simulink model "tank_based_bi_teleop_pf"  (R2020b)
settings: Solver=VariableStepAuto  StartTime=0.0  StopTime=4.0  RelTol=1e-3
values from neighbouring files (symbols this model uses):
  A = 1    [four_channel_bilateral_teleoperation_kalman_params.m]    (also in four_channel_bilateral_teleoperation_params.m; kalman_test.m = [1 Ts Ts^2/2; 0 1 Ts; 0 0 1]; recursive_estimation.m = [1 Ts Ts^2/2; 0 1 Ts; 0 0 1]; scattering_based_bi_teleop_pf_kalman_params.m)
  Be = 100    [four_channel_bilateral_teleoperation_architecture_params.m]    (also in four_channel_bilateral_teleoperation_kalman_params.m = 0; four_channel_bilateral_teleoperation_params.m = 0; scattering_based_bi_teleop_pf_kalman_params.m = 10; scattering_based_bi_teleop_pf_params.m = 10)
  Bh = 70    [four_channel_bilateral_teleoperation_architecture_params.m]    (also in four_channel_bilateral_teleoperation_kalman_params.m; four_channel_bilateral_teleoperation_params.m; scattering_based_bi_teleop_pf_kalman_params.m = 1.5; scattering_based_bi_teleop_pf_params.m = 1.5)
  Bm = 1    [four_channel_bilateral_teleoperation_architecture_params.m]    (also in four_channel_bilateral_teleoperation_kalman_params.m = 0.8; four_channel_bilateral_teleoperation_params.m = 0.8; scattering_based_bi_teleop_pf_kalman_params.m = 0; scattering_based_bi_teleop_pp_kalman_params.m = 15)
  Bs = 1    [four_channel_bilateral_teleoperation_architecture_params.m]    (also in four_channel_bilateral_teleoperation_kalman_params.m = 3.2; four_channel_bilateral_teleoperation_params.m = 3.2; scattering_based_bi_teleop_pf_kalman_params.m = 40; scattering_based_bi_teleop_pf_params.m = 3)
  Dh = 500    [four_channel_bilateral_teleoperation_kalman_params.m]    (also in four_channel_bilateral_teleoperation_params.m = 100; scattering_based_bi_teleop_pf_kalman_params.m = 0; scattering_based_bi_teleop_pf_params.m = 17; scattering_based_bi_teleop_pp_kalman_params.m = 0)
  Dm = 5    [four_channel_bilateral_teleoperation_architecture_params.m]    (also in four_channel_bilateral_teleoperation_kalman_params.m = 0; four_channel_bilateral_teleoperation_params.m = 0; scattering_based_bi_teleop_pf_kalman_params.m = 0; scattering_based_bi_teleop_pf_params.m = 0)
  Ds = 10    [four_channel_bilateral_teleoperation_architecture_params.m]    (also in four_channel_bilateral_teleoperation_kalman_params.m = 0; four_channel_bilateral_teleoperation_params.m = 0; scattering_based_bi_teleop_pf_kalman_params.m = 0; scattering_based_bi_teleop_pf_params.m = 0)
  Fc = 1    [four_channel_bilateral_teleoperation_kalman_params.m]    (also in four_channel_bilateral_teleoperation_params.m; kalman_test.m = 10; scattering_based_bi_teleop_pf_kalman_params.m = 0.1; scattering_based_bi_teleop_pf_params.m)
  Fip = 1    [four_channel_bilateral_teleoperation_kalman_params.m]    (also in four_channel_bilateral_teleoperation_params.m; scattering_based_bi_teleop_pf_kalman_params.m = 5; scattering_based_bi_teleop_pf_params.m; scattering_based_bi_teleop_pp_kalman_params.m = 5)
  Je = 0    [four_channel_bilateral_teleoperation_architecture_params.m]    (also in four_channel_bilateral_teleoperation_kalman_params.m; four_channel_bilateral_teleoperation_params.m; scattering_based_bi_teleop_pf_kalman_params.m; scattering_based_bi_teleop_pf_params.m)
  Jh = 0.5    [four_channel_bilateral_teleoperation_architecture_params.m]    (also in four_channel_bilateral_teleoperation_kalman_params.m; four_channel_bilateral_teleoperation_params.m; scattering_based_bi_teleop_pf_kalman_params.m = 0; scattering_based_bi_teleop_pf_params.m = 0.05)
  Ke = 200    [four_channel_bilateral_teleoperation_architecture_params.m]    (also in four_channel_bilateral_teleoperation_kalman_params.m = 50; four_channel_bilateral_teleoperation_params.m = 50; scattering_based_bi_teleop_pf_kalman_params.m; scattering_based_bi_teleop_pf_params.m)
  Kh = 2000    [four_channel_bilateral_teleoperation_architecture_params.m]    (also in four_channel_bilateral_teleoperation_kalman_params.m; four_channel_bilateral_teleoperation_params.m; scattering_based_bi_teleop_pf_kalman_params.m = 1; scattering_based_bi_teleop_pf_params.m = 0)
  Km = 1    [four_channel_bilateral_teleoperation_architecture_params.m]    (also in four_channel_bilateral_teleoperation_kalman_params.m; four_channel_bilateral_teleoperation_params.m; scattering_based_bi_teleop_pf_kalman_params.m = 0; scattering_based_bi_teleop_pp_kalman_params.m = 10)
  Ks = 1    [four_channel_bilateral_teleoperation_architecture_params.m]    (also in four_channel_bilateral_teleoperation_kalman_params.m = 4; four_channel_bilateral_teleoperation_params.m = 4; scattering_based_bi_teleop_pf_kalman_params.m = 50; scattering_based_bi_teleop_pf_params.m = 110)
  Mm = 0.5    [four_channel_bilateral_teleoperation_architecture_params.m]    (also in four_channel_bilateral_teleoperation_kalman_params.m; four_channel_bilateral_teleoperation_params.m; scattering_based_bi_teleop_pf_kalman_params.m; scattering_based_bi_teleop_pf_params.m)
  Ms = 2    [four_channel_bilateral_teleoperation_architecture_params.m]    (also in four_channel_bilateral_teleoperation_kalman_params.m; four_channel_bilateral_teleoperation_params.m; scattering_based_bi_teleop_pf_kalman_params.m; scattering_based_bi_teleop_pf_params.m)
  Ph = 2000    [four_channel_bilateral_teleoperation_kalman_params.m]    (also in four_channel_bilateral_teleoperation_params.m = 20100; scattering_based_bi_teleop_pf_kalman_params.m = 5; scattering_based_bi_teleop_pf_params.m = 23; scattering_based_bi_teleop_pp_kalman_params.m = 6)
  Ts = 0.001    [four_channel_bilateral_teleoperation_kalman_params.m]    (also in four_channel_bilateral_teleoperation_params.m; kalman_test.m; recursive_estimation.m; scattering_based_bi_teleop_pf_kalman_params.m)
undefined symbols (not defined in the file or in its folder): tau
libraries: simulink x2
settings Model: Creator=anuj  LastModifiedBy=filippo

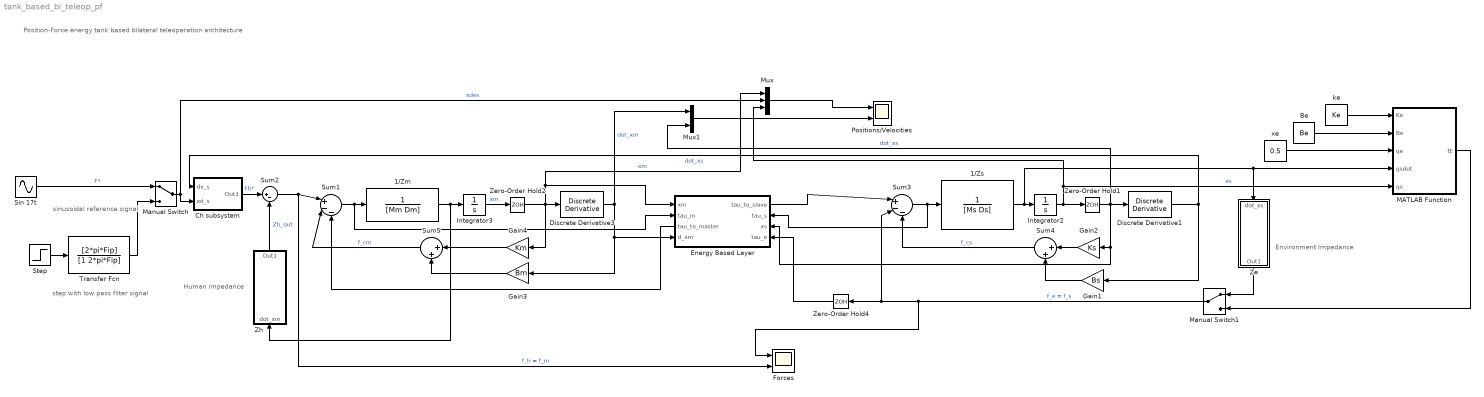
== system tank_based_bi_teleop_pf ==
  note: Position-Force energy tank based bilateral teleoperation architecture
  note: Environment Impedance
  note: Human impedance
  note: sinusoidal reference signal
  note: step with low pass filter signal
  1/Zm : TransferFcn  Denominator=[Mm Dm]
  1/Zs : TransferFcn  Denominator=[Ms Ds]
  Be : Constant  Value=Be
  Ch subsystem : Subsystem
  Discrete Derivative1 : simulink/Discrete/Discrete Derivative  gainval=1.0  ICPrevScaledInput=0.0  OutMin=[]  OutMax=[]  OutDataType=fixdt(1, 16)  OutScaling=2^-10  DoSatur=off
  Discrete Derivative3 : simulink/Discrete/Discrete Derivative  gainval=1.0  ICPrevScaledInput=0.0  OutMin=[]  OutMax=[]  OutDataType=fixdt(1, 16)  OutScaling=2^-10  DoSatur=off
  Energy Based Layer : Subsystem
      settings: PortSchema="{\"entries\":[{\"content\":{\"sides\":[{\"content\":{\"connectorIds\":[\"In1\",\"In2\",\"Out2\",\"In3\"]},\"type\":\"ConnectorPlacement.EquallySpacedRectSide\",\"uuid\":\"721fd75b-d64f-459b-a3fd-bbe3848745a1\"},{\"content\":{\"connectorIds\":[\"Out1\",\"In4\",\"In5\",\"In6\"],\"side\":\"RIGHT\"},\"type\":\"ConnectorPlacement.EquallySpacedRectSide\",\"uuid\":\"fbbe53d8-b5f9-4b89-bc3e-da0a725f4cb9\"},{\"content\":{\"connectorIds\":[],\"side\":\"TOP\"},\"type\":\"ConnectorPlacement.EquallySpacedRectSide\",\"uuid\":\"8cd4d438-c323-4c6b-8da9-ae64782b16ea\"},{\"content\":{\"connectorIds\":[],\"side\":\"HIDDEN\"},\"type\":\"ConnectorPlacement.EquallySpacedRectSide\",\"uuid\":\"3c4adbce-c957-4479-b649-6006afc34fa2\"}]},\"type\":\"ConnectorPlacement.EquallySpacedConnector\",\"uuid\":\"ae1c0201-3e75-47b3-8045-db2a4ffaac12\"}],\"packageUris\":[\"http://schema.mathworks.com/mf0/Connector/R2020b\"],\"version\":\"1.0\"}"
  Forces : Scope  NumInputPorts=2
  Gain1 : Gain  Gain=Bs
  Gain2 : Gain  Gain=Ks
  Gain3 : Gain  Gain=Bm
  Gain4 : Gain  Gain=Km
  Integrator2 : Integrator
  Integrator3 : Integrator
  MATLAB Function : MATLAB Function  TreatAsAtomicUnit=on
  Manual Switch : ManualSwitch
  Manual Switch1 : ManualSwitch
  Mux : Mux  Inputs=3
  Mux1 : Mux  Inputs=2
  Positions/Velocities : Scope  NumInputPorts=2
  Sin 17t : Sin  Amplitude=A  Frequency=2*pi*Fc  SampleTime=0
  Step : Step  After=A  SampleTime=0
  Sum1 : Sum  Inputs=|+--
  Sum2 : Sum  Inputs=|+-
  Sum3 : Sum  Inputs=|+--
  Sum4 : Sum  Inputs=|++
  Sum5 : Sum  Inputs=|++
  Transfer Fcn : TransferFcn  Numerator=[2*pi*Fip]  Denominator=[1 2*pi*Fip]
  Ze : Subsystem
  Zero-Order Hold1 : ZeroOrderHold  SampleTime=Ts
  Zero-Order Hold2 : ZeroOrderHold  SampleTime=Ts
  Zero-Order Hold4 : ZeroOrderHold  SampleTime=Ts
  Zh : Subsystem
  ke : Constant  Value=Ke
  xe : Constant  Value=0.5
  wires:
  Sum2/1 -> Forces/2, Sum1/1  "f_h = f_m"
  1/Zm/1 -> Integrator3/1, Zh/1(dot_xm)
  Sum1/1 -> Energy Based Layer/2(tau_m), 1/Zm/1
  Energy Based Layer/2(tau_to_master) -> Sum1/3
  Sum3/1 -> Energy Based Layer/4(tau_s), 1/Zs/1
  Manual Switch1/1 -> Forces/1, Sum3/2, Zero-Order Hold4/1  "f_e = f_s"
  Be/1 -> MATLAB Function/2(Be)
  xe/1 -> MATLAB Function/3(qe)
  ke/1 -> MATLAB Function/1(Ke)
  Transfer Fcn/1 -> Manual Switch/2
  Step/1 -> Transfer Fcn/1
  Sin 17t/1 -> Manual Switch/1  "F*"
  Energy Based Layer/1(tau_to_slave) -> Sum3/1
  Zh/1(Out1) -> Sum2/2  "Zh_out"
  Sum5/1 -> Sum1/2  "f_cm"
  Sum4/1 -> Sum3/3  "f_cs"
  Discrete Derivative1/1 -> Gain1/1, Ch subsystem/1(dx_s)  "dot_xs"
  1/Zs/1 -> Integrator2/1, Ze/1(dot_xs), MATLAB Function/4(qsdot)
  Integrator2/1 -> Zero-Order Hold1/1, Mux/3, MATLAB Function/5(qs)  "xs"
  Gain2/1 -> Sum4/1
  Gain1/1 -> Sum4/2
  Zero-Order Hold1/1 -> Mux1/2, Gain2/1, Energy Based Layer/5(xs), Discrete Derivative1/1  "dot_xs"
  Integrator3/1 -> Zero-Order Hold2/1  "xm"
  Gain4/1 -> Sum5/1
  Gain3/1 -> Sum5/2
  Discrete Derivative3/1 -> Energy Based Layer/3(d_xm), Gain3/1, Mux1/1  "dot_xm"
  Zero-Order Hold2/1 -> Energy Based Layer/1(xm), Mux/1, Gain4/1, Discrete Derivative3/1  "xm"
  Zero-Order Hold4/1 -> Energy Based Layer/6(tau_e)
  Ze/1(Out1) -> Manual Switch1/1
  MATLAB Function/1(fE) -> Manual Switch1/2
  Mux1/1 -> Positions/Velocities/2
  Mux/1 -> Positions/Velocities/1
  Manual Switch/1 -> Mux/2, Ch subsystem/2(xd_s)  "xdes"
  Ch subsystem/1(Out1) -> Sum2/1  "Fh*"

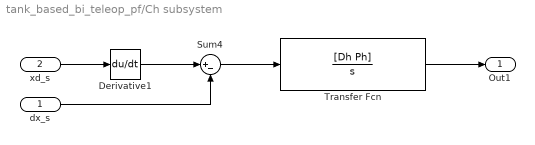
== system tank_based_bi_teleop_pf/Ch subsystem ==
  dx_s : Inport
  xd_s : Inport  Port=2
  Derivative1 : Derivative
  Sum4 : Sum  Inputs=|+-
  Transfer Fcn : TransferFcn  Numerator=[Dh Ph]  Denominator=[1 0]
  Out1 : Outport
  wires:
  dx_s/1 -> Sum4/2
  Derivative1/1 -> Sum4/1
  xd_s/1 -> Derivative1/1
  Sum4/1 -> Transfer Fcn/1
  Transfer Fcn/1 -> Out1/1

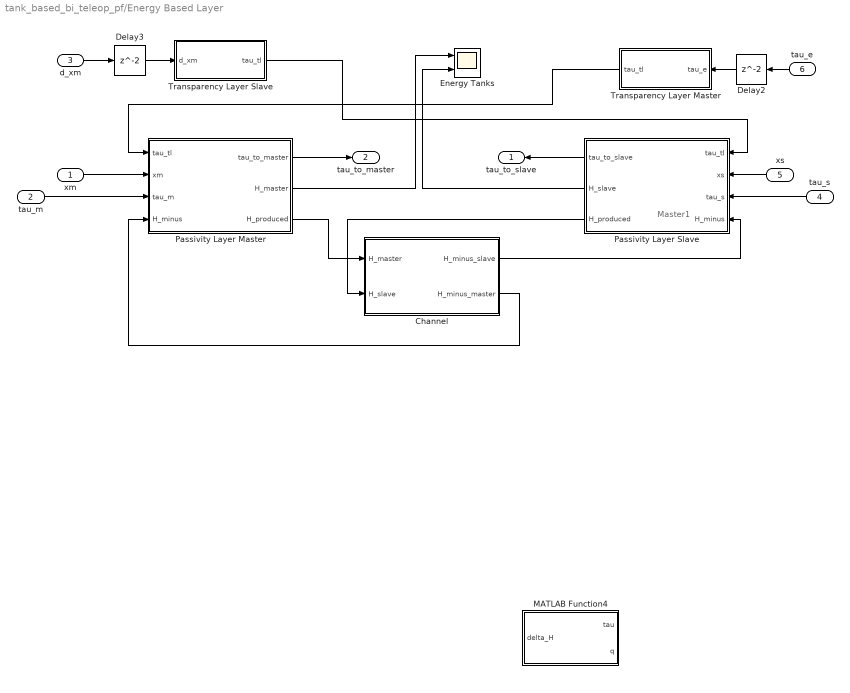
== system tank_based_bi_teleop_pf/Energy Based Layer ==
  note: Master1
  xm : Inport
  tau_m : Inport  Port=2
  d_xm : Inport  Port=3
  tau_s : Inport  Port=4
  xs : Inport  Port=5
  tau_e : Inport  Port=6
  Channel : Subsystem
  Delay2 : Delay
  Delay3 : Delay
  Energy Tanks : Scope  NumInputPorts=2
  MATLAB Function4 : MATLAB Function  TreatAsAtomicUnit=on
  Passivity Layer Master : Subsystem
  "Passivity Layer Slave " : Subsystem
  Transparency Layer Master : Subsystem
  Transparency Layer Slave : Subsystem
  tau_to_slave : Outport
  tau_to_master : Outport  Port=2
  wires:
  tau_e/1 -> Delay2/1
  Delay2/1 -> Transparency Layer Master/1(tau_e)
  d_xm/1 -> Delay3/1
  Delay3/1 -> Transparency Layer Slave/1(d_xm)
  tau_m/1 -> Passivity Layer Master/3(tau_m)
  xm/1 -> Passivity Layer Master/2(xm)
  tau_s/1 -> "Passivity Layer Slave "/3(tau_s)
  xs/1 -> "Passivity Layer Slave "/2(xs)
  "Passivity Layer Slave "/1(tau_to_slave) -> tau_to_slave/1
  Passivity Layer Master/1(tau_to_master) -> tau_to_master/1
  Passivity Layer Master/2(H_master) -> Energy Tanks/1
  "Passivity Layer Slave "/2(H_slave) -> Energy Tanks/2
  Passivity Layer Master/3(H_produced) -> Channel/1(H_master)
  "Passivity Layer Slave "/3(H_produced) -> Channel/2(H_slave)
  Channel/1(H_minus_slave) -> "Passivity Layer Slave "/4(H_minus)
  Channel/2(H_minus_master) -> Passivity Layer Master/4(H_minus)
  Transparency Layer Slave/1(tau_tl) -> "Passivity Layer Slave "/1(tau_tl)
  Transparency Layer Master/1(tau_tl) -> Passivity Layer Master/1(tau_tl)

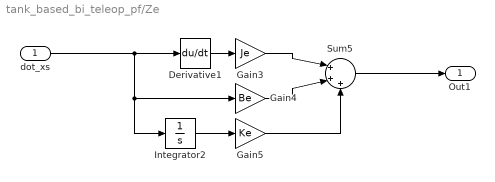
== system tank_based_bi_teleop_pf/Ze ==
  dot_xs : Inport
  Derivative1 : Derivative
  Gain3 : Gain  Gain=Je
  Gain4 : Gain  Gain=Be
  Gain5 : Gain  Gain=Ke
  Integrator2 : Integrator
  Sum5 : Sum  Inputs=|+++
  Out1 : Outport
  wires:
  Gain4/1 -> Sum5/2
  Gain3/1 -> Sum5/1
  Gain5/1 -> Sum5/3
  Sum5/1 -> Out1/1
  Integrator2/1 -> Gain5/1
  dot_xs/1 -> Integrator2/1, Gain4/1, Derivative1/1
  Derivative1/1 -> Gain3/1

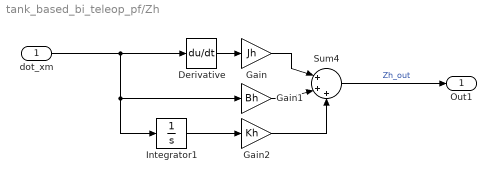
== system tank_based_bi_teleop_pf/Zh ==
  dot_xm : Inport
  Derivative : Derivative
  Gain : Gain  Gain=Jh
  Gain1 : Gain  Gain=Bh
  Gain2 : Gain  Gain=Kh
  Integrator1 : Integrator
  Sum4 : Sum  Inputs=|+++
  Out1 : Outport
  wires:
  Derivative/1 -> Gain/1
  Integrator1/1 -> Gain2/1
  Gain2/1 -> Sum4/3
  Gain1/1 -> Sum4/2
  Gain/1 -> Sum4/1
  Sum4/1 -> Out1/1  "Zh_out"
  dot_xm/1 -> Gain1/1, Integrator1/1, Derivative/1

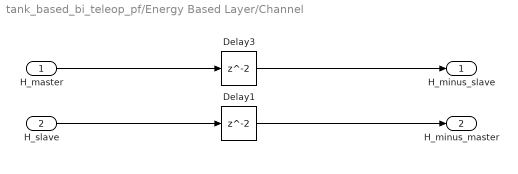
== system tank_based_bi_teleop_pf/Energy Based Layer/Channel ==
  H_master : Inport
  H_slave : Inport  Port=2
  Delay1 : Delay
  Delay3 : Delay
  H_minus_slave : Outport
  H_minus_master : Outport  Port=2
  wires:
  H_master/1 -> Delay3/1
  H_slave/1 -> Delay1/1
  Delay3/1 -> H_minus_slave/1
  Delay1/1 -> H_minus_master/1

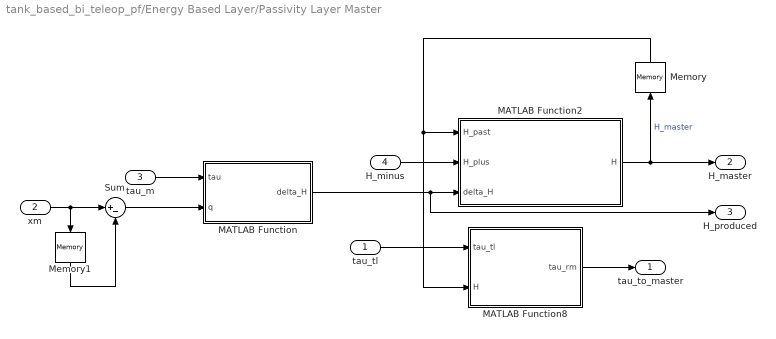
== system tank_based_bi_teleop_pf/Energy Based Layer/Passivity Layer Master ==
  tau_tl : Inport
  xm : Inport  Port=2
  tau_m : Inport  Port=3
  H_minus : Inport  Port=4
  MATLAB Function : MATLAB Function  TreatAsAtomicUnit=on
  MATLAB Function2 : MATLAB Function  TreatAsAtomicUnit=on
  MATLAB Function8 : MATLAB Function  TreatAsAtomicUnit=on
  Memory : Memory
  Memory1 : Memory
  Sum : Sum  Inputs=|+-
  tau_to_master : Outport
  H_master : Outport  Port=2
  H_produced : Outport  Port=3
  wires:
  MATLAB Function2/1(H) -> H_master/1, Memory/1  "H_master"
  tau_m/1 -> MATLAB Function/1(tau)
  Memory/1 -> MATLAB Function8/2(H), MATLAB Function2/1(H_past)
  MATLAB Function/1(delta_H) -> H_produced/1, MATLAB Function2/3(delta_H)
  xm/1 -> Sum/1, Memory1/1
  tau_tl/1 -> MATLAB Function8/1(tau_tl)
  H_minus/1 -> MATLAB Function2/2(H_plus)
  Memory1/1 -> Sum/2
  Sum/1 -> MATLAB Function/2(q)
  MATLAB Function8/1(tau_rm) -> tau_to_master/1

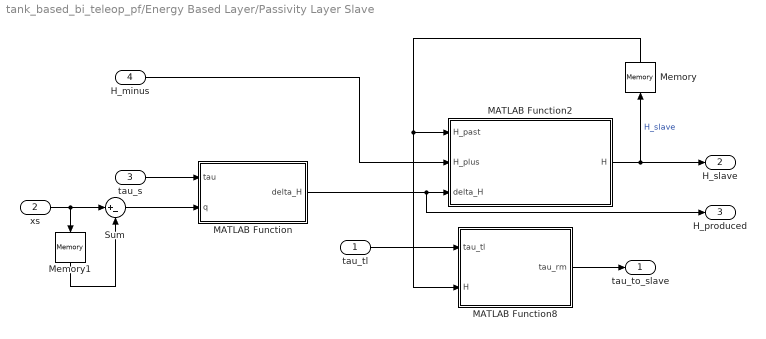
== system tank_based_bi_teleop_pf/Energy Based Layer/Passivity Layer Slave  ==
  tau_tl : Inport
  xs : Inport  Port=2
  tau_s : Inport  Port=3
  H_minus : Inport  Port=4
  MATLAB Function : MATLAB Function  TreatAsAtomicUnit=on
  MATLAB Function2 : MATLAB Function  TreatAsAtomicUnit=on
  MATLAB Function8 : MATLAB Function  TreatAsAtomicUnit=on
  Memory : Memory
  Memory1 : Memory
  Sum : Sum  Inputs=|+-
  tau_to_slave : Outport
  H_slave : Outport  Port=2
  H_produced : Outport  Port=3
  wires:
  MATLAB Function2/1(H) -> H_slave/1, Memory/1  "H_slave"
  tau_s/1 -> MATLAB Function/1(tau)
  Memory/1 -> MATLAB Function8/2(H), MATLAB Function2/1(H_past)
  MATLAB Function/1(delta_H) -> H_produced/1, MATLAB Function2/3(delta_H)
  MATLAB Function8/1(tau_rm) -> tau_to_slave/1
  tau_tl/1 -> MATLAB Function8/1(tau_tl)
  H_minus/1 -> MATLAB Function2/2(H_plus)
  Sum/1 -> MATLAB Function/2(q)
  xs/1 -> Sum/1, Memory1/1
  Memory1/1 -> Sum/2

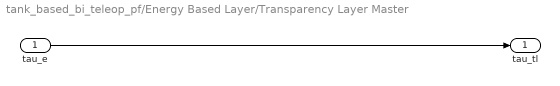
== system tank_based_bi_teleop_pf/Energy Based Layer/Transparency Layer Master ==
  tau_e : Inport
  tau_tl : Outport
  wires:
  tau_e/1 -> tau_tl/1

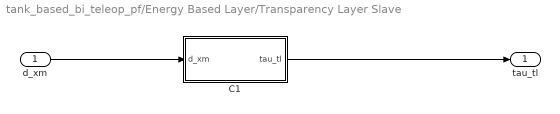
== system tank_based_bi_teleop_pf/Energy Based Layer/Transparency Layer Slave ==
  d_xm : Inport
  C1 : Subsystem
  tau_tl : Outport
  wires:
  d_xm/1 -> C1/1(d_xm)
  C1/1(tau_tl) -> tau_tl/1

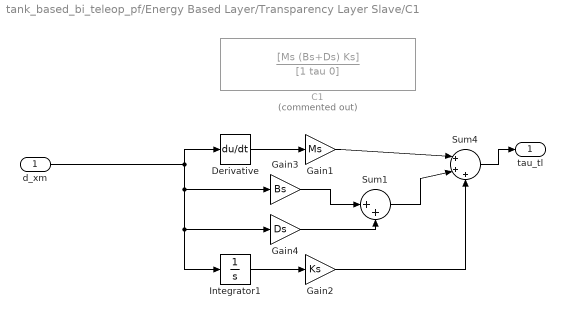
== system tank_based_bi_teleop_pf/Energy Based Layer/Transparency Layer Slave/C1 ==
  d_xm : Inport
  C1 : TransferFcn  Commented=on  Numerator=[Ms (Bs+Ds) Ks]  Denominator=[1 tau 0]
  Derivative : Derivative
  Gain1 : Gain  Gain=Ms
  Gain2 : Gain  Gain=Ks
  Gain3 : Gain  Gain=Bs
  Gain4 : Gain  Gain=Ds
  Integrator1 : Integrator
  Sum1 : Sum  Inputs=|++
  Sum4 : Sum  Inputs=|+++
  tau_tl : Outport
  wires:
  Sum4/1 -> tau_tl/1
  Gain1/1 -> Sum4/1
  Integrator1/1 -> Gain2/1
  d_xm/1 -> Derivative/1, Gain3/1, Integrator1/1, Gain4/1
  Gain2/1 -> Sum4/3
  Sum1/1 -> Sum4/2
  Gain4/1 -> Sum1/2
  Gain3/1 -> Sum1/1
  Derivative/1 -> Gain1/1

== matlab function tank_based_bi_teleop_pf/Energy Based Layer/Passivity Layer Slave /MATLAB Function ==
  data: tau input; delta_H output; q input
function delta_H = delta_H(tau, q)
    delta_H = tau*q;
end

== matlab function tank_based_bi_teleop_pf/MATLAB Function ==
  data: Ke input; fE output; Be input; qe input; qsdot input; qs input
function fE = environment(Ke, Be, qe, qsdot, qs)
    if qs > qe
        fE = Ke * (qs - qe) + Be * qsdot; % Plot both contributions Ke and Be
    else
        fE = 0;
    end
end

== matlab function tank_based_bi_teleop_pf/Energy Based Layer/Passivity Layer Slave /MATLAB Function2 ==
  data: H output; H_past input; H_plus input; delta_H input
function H = EnergyTank(H_past, H_plus, delta_H)
    H = H_past + H_plus - delta_H;
end

== matlab function tank_based_bi_teleop_pf/Energy Based Layer/Passivity Layer Slave /MATLAB Function8 ==
  data: tau_tl input; tau_rm output; H input
function tau_rm = tau_saturation(tau_tl, H)
    tau_max1 = tau_tl;
    if H <= 0 
       tau_max1 = 0;
    end
    
    tau_rm = sign(tau_tl)*min(abs(tau_tl), tau_max1);
end

== matlab function tank_based_bi_teleop_pf/Energy Based Layer/MATLAB Function4 ==
  data: tau input; delta_H output; q input
function delta_H = delta_H(tau, q)
    delta_H = tau*q;
end

== matlab function tank_based_bi_teleop_pf/Energy Based Layer/Passivity Layer Master/MATLAB Function ==
  data: tau input; delta_H output; q input
function delta_H = delta_H(tau, q)
    delta_H = tau*q;
end

== matlab function tank_based_bi_teleop_pf/Energy Based Layer/Passivity Layer Master/MATLAB Function2 ==
  data: H output; H_past input; H_plus input; delta_H input
function H = EnergyTank(H_past, H_plus, delta_H)
    H = H_past + H_plus - delta_H;
end

== matlab function tank_based_bi_teleop_pf/Energy Based Layer/Passivity Layer Master/MATLAB Function8 ==
  data: tau_tl input; tau_rm output; H input
function tau_rm = tau_saturation(tau_tl, H)
    tau_max1 = tau_tl;
    if H <= 0 
       tau_max1 = 0;
    end
    
    tau_rm = sign(tau_tl)*min(abs(tau_tl), tau_max1);
end
